simulink model "lpv_modeling"  (R2022b)
settings: Solver=VariableStepAuto  StartTime=0.0  StopTime=10  RelTol=1e-3
undefined symbols (not defined in the file): B, C, D
libraries: cstblocks x4
settings Model: Creator=phatdo  LastModifiedBy=phatdo

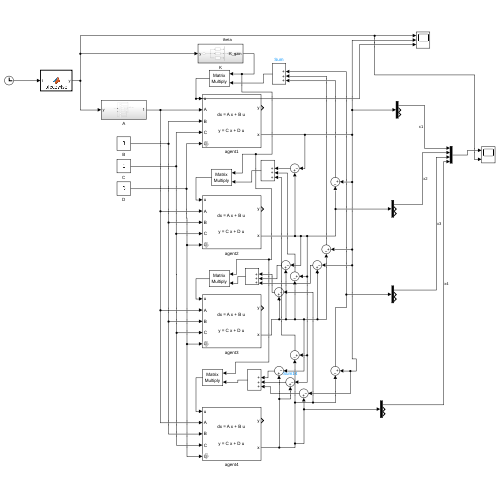
[thumbnail: Simulink's stored preview of the top-level diagram]
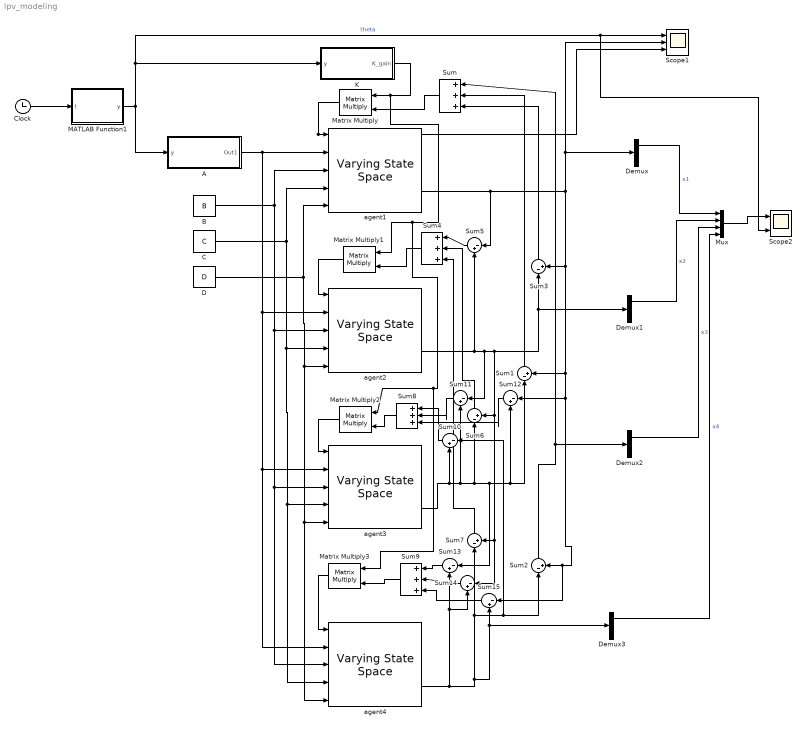
== system lpv_modeling ==
  A : Subsystem
  B : Constant  Value=B
  C : Constant  Value=C  VectorParams1D=off
  Clock : Clock
  D : Constant  Value=D  VectorParams1D=off
  Demux{,1..3} (4 alike) : Demux  Outputs=3
  K : Subsystem
  MATLAB Function1 : MATLAB Function  TreatAsAtomicUnit=on
  Matrix Multiply{,1..3} (4 alike) : Product  Multiplication=Matrix(*)
  Mux : Mux
  Scope1 : Scope  NumInputPorts=3
  Scope2 : Scope  NumInputPorts=2
  Sum{,4,8..9} (4 alike) : Sum  Inputs=|+++
  Sum{1..3,5..7,10..15} (12 alike) : Sum  Inputs=|-+
  agent1 : cstblocks/Linear Parameter Varying/Varying State Space  x0=[5;0;0]  xNames=''  OutputX=on  OutputDX=off
  agent2 : cstblocks/Linear Parameter Varying/Varying State Space  x0=[1;0;0]  xNames=''  OutputX=on  OutputDX=off
  agent3 : cstblocks/Linear Parameter Varying/Varying State Space  x0=[-3;0;0]  xNames=''  OutputX=on  OutputDX=off
  agent4 : cstblocks/Linear Parameter Varying/Varying State Space  x0=[-3;0;0]  xNames=''  OutputX=on  OutputDX=off
  wires:
  Clock/1 -> MATLAB Function1/1(t)
  MATLAB Function1/1(y) -> A/1(y), K/1(y), Scope2/2, Scope1/1  "theta"
  C/1 -> agent4/4, agent3/4, agent2/4, agent1/4
  B/1 -> agent4/3, agent3/3, agent2/3, agent1/3
  D/1 -> agent1/5, agent4/5, agent3/5, agent2/5
  A/1(Out1) -> agent4/2, agent3/2, agent2/2, agent1/2
  agent2/2 -> Sum5/2, Sum11/1, Sum14/1, Sum7/2, Sum6/2, Demux1/1, Sum3/1
  agent3/2 -> Sum10/2, Sum11/2, Sum6/1, Sum13/1, Sum12/2, Sum1/1
  agent4/2 -> Sum14/2, Sum13/2, Demux3/1, Sum15/2, Sum7/1, Sum10/1, Sum2/1
  agent1/2 -> Sum5/1, Demux/1, Scope1/2, Sum3/2, Sum1/2, Sum12/1, Sum15/1, Sum2/2
  Sum3/1 -> Sum/3
  Sum1/1 -> Sum/2
  Sum2/1 -> Demux2/1, Sum/1
  Sum/1 -> Matrix Multiply/2
  K/1(K_gain) -> Matrix Multiply3/1, Matrix Multiply2/1, Matrix Multiply1/1, Matrix Multiply/1
  Matrix Multiply/1 -> Scope1/3, agent1/1
  Matrix Multiply1/1 -> agent2/1
  Sum5/1 -> Sum4/1
  Sum6/1 -> Sum4/2
  Sum7/1 -> Sum4/3
  Sum4/1 -> Matrix Multiply1/2
  Sum8/1 -> Matrix Multiply2/2
  Sum9/1 -> Matrix Multiply3/2
  Matrix Multiply2/1 -> agent3/1
  Matrix Multiply3/1 -> agent4/1
  Sum10/1 -> Sum8/1
  Sum11/1 -> Sum8/2
  Sum12/1 -> Sum8/3
  Sum13/1 -> Sum9/1
  Sum14/1 -> Sum9/2
  Sum15/1 -> Sum9/3
  Demux/1 -> Mux/1  "x1"
  Demux1/1 -> Mux/2  "x2"
  Demux2/1 -> Mux/3  "x3"
  Demux3/1 -> Mux/4  "x4"
  Mux/1 -> Scope2/1

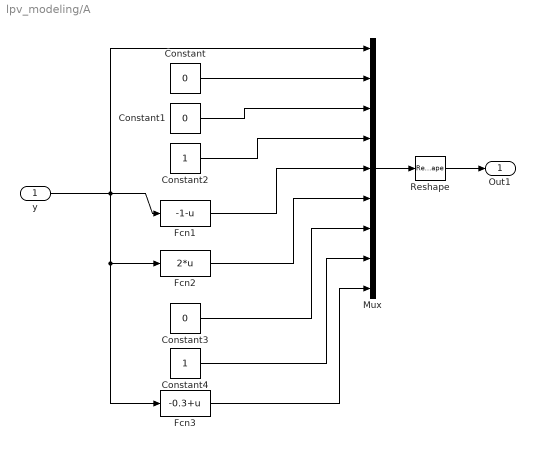
== system lpv_modeling/A ==
  y : Inport
  Constant : Constant  Value=0
  Constant1 : Constant  Value=0
  Constant2 : Constant
  Constant3 : Constant  Value=0
  Constant4 : Constant
  Fcn1 : Fcn  Expr=-1-u
  Fcn2 : Fcn  Expr=2*u
  Fcn3 : Fcn  Expr=-0.3+u
  Mux : Mux  Inputs=9
  Reshape : Reshape  OutputDimensionality=Customize  OutputDimensions=[3,3]
  Out1 : Outport
  wires:
  Mux/1 -> Reshape/1
  y/1 -> Fcn3/1, Fcn2/1, Fcn1/1, Mux/1
  Constant/1 -> Mux/2
  Constant1/1 -> Mux/3
  Constant2/1 -> Mux/4
  Fcn1/1 -> Mux/5
  Fcn2/1 -> Mux/6
  Constant3/1 -> Mux/7
  Constant4/1 -> Mux/8
  Reshape/1 -> Out1/1
  Fcn3/1 -> Mux/9

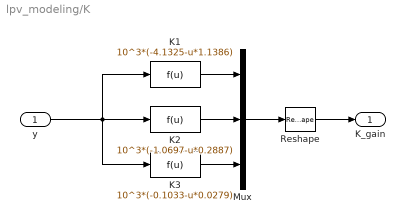
== system lpv_modeling/K ==
  y : Inport
  K1 : Fcn  Expr=10^3*(-4.1325-u*1.1386)
  K2 : Fcn  Expr=10^3*(-1.0697-u*0.2887)
  K3 : Fcn  Expr=10^3*(-0.1033-u*0.0279)
  Mux : Mux  Inputs=3
  Reshape : Reshape  OutputDimensionality=Customize  OutputDimensions=[1,3]
  K_gain : Outport
  wires:
  Mux/1 -> Reshape/1
  Reshape/1 -> K_gain/1
  K1/1 -> Mux/1
  K2/1 -> Mux/2
  K3/1 -> Mux/3
  y/1 -> K3/1, K1/1, K2/1

== matlab function lpv_modeling/MATLAB Function1 ==
  data: t input; y output
function y = piecewise(t)

if t <= 2
    y = 1.5;
elseif (t > 2) && (t <= 3)
    y = -1;
elseif (t > 3) && (t <= 5)
    y = 1.8;
elseif (t > 5) && (t <= 7)
    y = -1.5;
elseif (t > 7) && (t <= 9)
    y = 1.1;
else 
    y = -1.2;
end
